simulink model "nonLin_Model_std_V2"  (R2023b)
settings: Solver=ode23t  StartTime=0.0  StopTime=Tend  FixedStep=Ts  MaxStep=0.002  RelTol=1e-3
InitFcn:
  | sysParam = load("sysParam.mat");
  | load('./zz_temp/controlletTypeToUse.mat')
undefined symbols (not defined in the file): C, sysID
libraries: slpidlib x12, cstblocks x2
(part 2 of 2)

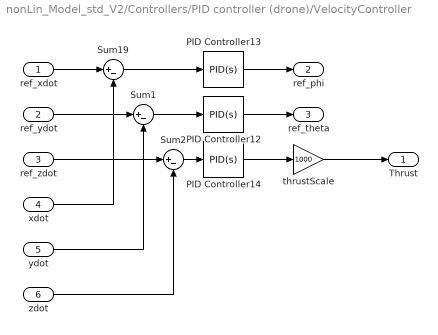
== system nonLin_Model_std_V2/Controllers/PID controller (drone)/VelocityController ==
  ref_xdot : Inport
  ref_ydot : Inport  Port=2
  ref_zdot : Inport  Port=3
  xdot : Inport  Port=4
  ydot : Inport  Port=5
  zdot : Inport  Port=6
  PID Controller12 : slpidlib/PID Controller  Controller=PID  Form=Parallel  TimeDomain=Continuous-time  UseExternalTs=off  SampleTime=-1  IntegratorMethod=Forward Euler  FilterMethod=Forward Euler  ControllerParametersSource=internal  P=C.vel.ydot.Kp  I=C.vel.ydot.Ki  UseKiTs=off  D=C.vel.ydot.Kd  N=100  UseFilter=on  TunerSelectOption=Transfer Function Based (PID Tuner App)  InitialConditionSource=internal  InitialConditionForIntegrator=0  InitialConditionForFilter=0  DifferentiatorICPrevScaledInput=0  ExternalReset=none  TrackingMode=off  Kt=1  LimitOutput=off  SatLimitsSource=internal  UpperSaturationLimit=inf  LowerSaturationLimit=-inf  LinearizeAsGain=on  AntiWindupMode=none  Kb=1  LimitIntegrator=off  UpperIntegratorSaturationLimit=inf  LowerIntegratorSaturationLimit=-inf  POutMin=[]  POutMax=[]  IOutMin=[]  IOutMax=[]  DOutMin=[]  DOutMax=[]  NOutMin=[]  NOutMax=[]  SumOutMin=[]  SumOutMax=[]  SaturationOutMin=[]  SaturationOutMax=[]  PParamMin=[]  PParamMax=[]  IParamMin=[]  IParamMax=[]  DParamMin=[]  DParamMax=[]  NParamMin=[]  NParamMax=[]  KbParamMin=[]  KbParamMax=[]  KtParamMin=[]  KtParamMax=[]  KbOutMin=[]  KbOutMax=[]  KtOutMin=[]  KtOutMax=[]  IntegratorOutMin=[]  IntegratorOutMax=[]  FilterOutMin=[]  FilterOutMax=[]  SumI1OutMin=[]  SumI1OutMax=[]  SumI2OutMin=[]  SumI2OutMax=[]  SumI3OutMin=[]  SumI3OutMax=[]  SumI4OutMin=[]  SumI4OutMax=[]  SumDOutMin=[]  SumDOutMax=[]  DifferentiatorOutMin=[]  DifferentiatorOutMax=[]  FilterDiffOutCoefMin=[]  FilterDiffOutCoefMax=[]  ReciprocalOutMin=[]  ReciprocalOutMax=[]  SumDenOutMin=[]  SumDenOutMax=[]  SumNumOutMin=[]  SumNumOutMax=[]  DivideOutMin=[]  DivideOutMax=[]  UdiffTsProdOutMin=[]  UdiffTsProdOutMax=[]  NTsProdOutMin=[]  NTsProdOutMax=[]  UintegralTsProdOutMin=[]  UintegralTsProdOutMax=[]  UngainTsProdOutMin=[]  UngainTsProdOutMax=[]  ClampingZeroOutDataTypeStr=Inherit: Inherit via back propagation  ClampingZeroOutMin=[]  ClampingZeroOutMax=[]  FilterDenConstantOutDataTypeStr=Inherit: Inherit via back propagation  FilterDenConstantOutMin=[]  FilterDenConstantOutMax=[]  PCopyOutDataTypeStr=Inherit: Inherit via back propagation  PCopyOutMin=[]  PCopyOutMax=[]  NCopyOutDataTypeStr=Inherit: Inherit via back propagation  NCopyOutMin=[]  NCopyOutMax=[]  IntegratorContinuousStateAttributes=''  IntegratorStateMustResolveToSignalObject=off  IntegratorRTWStateStorageClass=Auto  FilterContinuousStateAttributes=''  FilterStateMustResolveToSignalObject=off  FilterRTWStateStorageClass=Auto  ParallelPVariant=InternalParameters  IdealPVariant=Disabled  IVariant=InternalParameters  DVariant=InternalParameters  IntegratorVariant=Continuous  SatVariant=Disabled  AWVariant=Passthrough  PCopyVariant=Disabled  TRVariant=Disabled  FdbkBlocksVariant=Forward  IdealPFdbkVariant=Disabled  SatFdbkVariant=Disabled  DerivativeFilterVariant=ContFilter  NVariant=InternalParameters  NCopyVariant=Disabled  FilterICVariant=InternalICsFilter  IntegratorICVariant=InternalICs  ExternalResetVariant=Disabled  TRSumVariant=Passthrough  SumFdbkVariant=Disabled  SumVariant=Sum_PID  TsampFilterVariant=InternalTs  TsampNgainVariant=Passthrough  TsampIntegralVariant=Disabled_SignalSpec  ExternalSaturationOutDataTypeStr=Inherit: Same as second input
  PID Controller13 : slpidlib/PID Controller  Controller=PID  Form=Parallel  TimeDomain=Continuous-time  UseExternalTs=off  SampleTime=-1  IntegratorMethod=Forward Euler  FilterMethod=Forward Euler  ControllerParametersSource=internal  P=C.vel.xdot.Kp  I=C.vel.xdot.Ki  UseKiTs=off  D=C.vel.xdot.Kd  N=100  UseFilter=on  TunerSelectOption=Transfer Function Based (PID Tuner App)  InitialConditionSource=internal  InitialConditionForIntegrator=0  InitialConditionForFilter=0  DifferentiatorICPrevScaledInput=0  ExternalReset=none  TrackingMode=off  Kt=1  LimitOutput=off  SatLimitsSource=internal  UpperSaturationLimit=inf  LowerSaturationLimit=-inf  LinearizeAsGain=on  AntiWindupMode=none  Kb=1  LimitIntegrator=off  UpperIntegratorSaturationLimit=inf  LowerIntegratorSaturationLimit=-inf  POutMin=[]  POutMax=[]  IOutMin=[]  IOutMax=[]  DOutMin=[]  DOutMax=[]  NOutMin=[]  NOutMax=[]  SumOutMin=[]  SumOutMax=[]  SaturationOutMin=[]  SaturationOutMax=[]  PParamMin=[]  PParamMax=[]  IParamMin=[]  IParamMax=[]  DParamMin=[]  DParamMax=[]  NParamMin=[]  NParamMax=[]  KbParamMin=[]  KbParamMax=[]  KtParamMin=[]  KtParamMax=[]  KbOutMin=[]  KbOutMax=[]  KtOutMin=[]  KtOutMax=[]  IntegratorOutMin=[]  IntegratorOutMax=[]  FilterOutMin=[]  FilterOutMax=[]  SumI1OutMin=[]  SumI1OutMax=[]  SumI2OutMin=[]  SumI2OutMax=[]  SumI3OutMin=[]  SumI3OutMax=[]  SumI4OutMin=[]  SumI4OutMax=[]  SumDOutMin=[]  SumDOutMax=[]  DifferentiatorOutMin=[]  DifferentiatorOutMax=[]  FilterDiffOutCoefMin=[]  FilterDiffOutCoefMax=[]  ReciprocalOutMin=[]  ReciprocalOutMax=[]  SumDenOutMin=[]  SumDenOutMax=[]  SumNumOutMin=[]  SumNumOutMax=[]  DivideOutMin=[]  DivideOutMax=[]  UdiffTsProdOutMin=[]  UdiffTsProdOutMax=[]  NTsProdOutMin=[]  NTsProdOutMax=[]  UintegralTsProdOutMin=[]  UintegralTsProdOutMax=[]  UngainTsProdOutMin=[]  UngainTsProdOutMax=[]  ClampingZeroOutDataTypeStr=Inherit: Inherit via back propagation  ClampingZeroOutMin=[]  ClampingZeroOutMax=[]  FilterDenConstantOutDataTypeStr=Inherit: Inherit via back propagation  FilterDenConstantOutMin=[]  FilterDenConstantOutMax=[]  PCopyOutDataTypeStr=Inherit: Inherit via back propagation  PCopyOutMin=[]  PCopyOutMax=[]  NCopyOutDataTypeStr=Inherit: Inherit via back propagation  NCopyOutMin=[]  NCopyOutMax=[]  IntegratorContinuousStateAttributes=''  IntegratorStateMustResolveToSignalObject=off  IntegratorRTWStateStorageClass=Auto  FilterContinuousStateAttributes=''  FilterStateMustResolveToSignalObject=off  FilterRTWStateStorageClass=Auto  ParallelPVariant=InternalParameters  IdealPVariant=Disabled  IVariant=InternalParameters  DVariant=InternalParameters  IntegratorVariant=Continuous  SatVariant=Disabled  AWVariant=Passthrough  PCopyVariant=Disabled  TRVariant=Disabled  FdbkBlocksVariant=Forward  IdealPFdbkVariant=Disabled  SatFdbkVariant=Disabled  DerivativeFilterVariant=ContFilter  NVariant=InternalParameters  NCopyVariant=Disabled  FilterICVariant=InternalICsFilter  IntegratorICVariant=InternalICs  ExternalResetVariant=Disabled  TRSumVariant=Passthrough  SumFdbkVariant=Disabled  SumVariant=Sum_PID  TsampFilterVariant=InternalTs  TsampNgainVariant=Passthrough  TsampIntegralVariant=Disabled_SignalSpec  ExternalSaturationOutDataTypeStr=Inherit: Same as second input
  PID Controller14 : slpidlib/PID Controller  Controller=PID  Form=Parallel  TimeDomain=Continuous-time  UseExternalTs=off  SampleTime=-1  IntegratorMethod=Forward Euler  FilterMethod=Forward Euler  ControllerParametersSource=internal  P=C.vel.zdot.Kp  I=C.vel.zdot.Ki  UseKiTs=off  D=C.vel.zdot.Kd  N=100  UseFilter=on  TunerSelectOption=Transfer Function Based (PID Tuner App)  InitialConditionSource=internal  InitialConditionForIntegrator=0  InitialConditionForFilter=0  DifferentiatorICPrevScaledInput=0  ExternalReset=none  TrackingMode=off  Kt=1  LimitOutput=off  SatLimitsSource=internal  UpperSaturationLimit=inf  LowerSaturationLimit=-inf  LinearizeAsGain=on  AntiWindupMode=none  Kb=1  LimitIntegrator=off  UpperIntegratorSaturationLimit=inf  LowerIntegratorSaturationLimit=-inf  POutMin=[]  POutMax=[]  IOutMin=[]  IOutMax=[]  DOutMin=[]  DOutMax=[]  NOutMin=[]  NOutMax=[]  SumOutMin=[]  SumOutMax=[]  SaturationOutMin=[]  SaturationOutMax=[]  PParamMin=[]  PParamMax=[]  IParamMin=[]  IParamMax=[]  DParamMin=[]  DParamMax=[]  NParamMin=[]  NParamMax=[]  KbParamMin=[]  KbParamMax=[]  KtParamMin=[]  KtParamMax=[]  KbOutMin=[]  KbOutMax=[]  KtOutMin=[]  KtOutMax=[]  IntegratorOutMin=[]  IntegratorOutMax=[]  FilterOutMin=[]  FilterOutMax=[]  SumI1OutMin=[]  SumI1OutMax=[]  SumI2OutMin=[]  SumI2OutMax=[]  SumI3OutMin=[]  SumI3OutMax=[]  SumI4OutMin=[]  SumI4OutMax=[]  SumDOutMin=[]  SumDOutMax=[]  DifferentiatorOutMin=[]  DifferentiatorOutMax=[]  FilterDiffOutCoefMin=[]  FilterDiffOutCoefMax=[]  ReciprocalOutMin=[]  ReciprocalOutMax=[]  SumDenOutMin=[]  SumDenOutMax=[]  SumNumOutMin=[]  SumNumOutMax=[]  DivideOutMin=[]  DivideOutMax=[]  UdiffTsProdOutMin=[]  UdiffTsProdOutMax=[]  NTsProdOutMin=[]  NTsProdOutMax=[]  UintegralTsProdOutMin=[]  UintegralTsProdOutMax=[]  UngainTsProdOutMin=[]  UngainTsProdOutMax=[]  ClampingZeroOutDataTypeStr=Inherit: Inherit via back propagation  ClampingZeroOutMin=[]  ClampingZeroOutMax=[]  FilterDenConstantOutDataTypeStr=Inherit: Inherit via back propagation  FilterDenConstantOutMin=[]  FilterDenConstantOutMax=[]  PCopyOutDataTypeStr=Inherit: Inherit via back propagation  PCopyOutMin=[]  PCopyOutMax=[]  NCopyOutDataTypeStr=Inherit: Inherit via back propagation  NCopyOutMin=[]  NCopyOutMax=[]  IntegratorContinuousStateAttributes=''  IntegratorStateMustResolveToSignalObject=off  IntegratorRTWStateStorageClass=Auto  FilterContinuousStateAttributes=''  FilterStateMustResolveToSignalObject=off  FilterRTWStateStorageClass=Auto  ParallelPVariant=InternalParameters  IdealPVariant=Disabled  IVariant=InternalParameters  DVariant=InternalParameters  IntegratorVariant=Continuous  SatVariant=Disabled  AWVariant=Passthrough  PCopyVariant=Disabled  TRVariant=Disabled  FdbkBlocksVariant=Forward  IdealPFdbkVariant=Disabled  SatFdbkVariant=Disabled  DerivativeFilterVariant=ContFilter  NVariant=InternalParameters  NCopyVariant=Disabled  FilterICVariant=InternalICsFilter  IntegratorICVariant=InternalICs  ExternalResetVariant=Disabled  TRSumVariant=Passthrough  SumFdbkVariant=Disabled  SumVariant=Sum_PID  TsampFilterVariant=InternalTs  TsampNgainVariant=Passthrough  TsampIntegralVariant=Disabled_SignalSpec  ExternalSaturationOutDataTypeStr=Inherit: Same as second input
  Sum1 : Sum  Inputs=|+-
  Sum19 : Sum  Inputs=|+-
  Sum2 : Sum  Inputs=|+-
  thrustScale : Gain  Gain=1000
  Thrust : Outport
  ref_phi : Outport  Port=2
  ref_theta : Outport  Port=3
  wires:
  xdot/1 -> Sum19/2
  Sum19/1 -> PID Controller13/1
  Sum1/1 -> PID Controller12/1
  zdot/1 -> Sum2/2
  Sum2/1 -> PID Controller14/1
  ydot/1 -> Sum1/2
  ref_xdot/1 -> Sum19/1
  ref_ydot/1 -> Sum1/1
  ref_zdot/1 -> Sum2/1
  PID Controller14/1 -> thrustScale/1
  PID Controller12/1 -> ref_theta/1
  PID Controller13/1 -> ref_phi/1
  thrustScale/1 -> Thrust/1

== matlab function nonLin_Model_std_V2/non-linear model/MATLAB Function ==
  data: u input; dx output; x input; type input; sys_param2 parameter
function dx= nonLinDrone(u,x,type, sys_param2)
    m = sys_param2.m;
    I = sys_param2.I;
    g = sys_param2.g;
    % invI = inv(I);
    invI = sys_param2.inv_I;
    L = sys_param2.L;

    dx = zeros(12,1);
    
    % Angle states for easier use
    phi   = x(7); 
    theta = x(8); 
    psi   = x(9);
    p     = x(10); 
    q     = x(11); 
    r     = x(12);

    % Rotation matrix
    R = rotation_matrix(phi, theta, psi);

    % x and xdot definition
    dx(1:3,1) = [x(4); x(5); x(6)];
    dx(4:6,1) = 1/m*([0;0;-m*g]+R*[0;0;u(1)]);

    multiplication_matrix_pqr = ([1 sin(phi)*tan(theta) cos(phi)*tan(theta);0 cos(phi) -sin(phi);0 sin(phi)/cos(theta) cos(phi)/cos(theta)]);

    dx(7:9,1) = multiplication_matrix_pqr*[p;q;r];
    dx(10:12,1) = invI * ([u(2); u(3); u(4)] - cross([x(10);x(11);x(12)],I*[x(10);x(11);x(12)]));

    switch type
        case 1
            %F only
            dx([1:2 4:5 7:12]) = zeros(1,10);
        case 2
            %Mx only
            dx([1:6 8:9 11:12]) = zeros(1,10);
        case 3
            %My only
            dx([1:7 9:10 12]) = zeros(1,10);
        case 4
            %Mz only
            dx([1:8 10:11]) = zeros(1,10);
    end

function R = rotation_matrix(phi, theta, psi)
    R_x = [1 0 0; 0 cos(phi) -sin(phi); 0 sin(phi) cos(phi)];
    R_y = [cos(theta) 0 sin(theta); 0 1 0; -sin(theta) 0 cos(theta)];
    R_z = [cos(psi) -sin(psi) 0; sin(psi) cos(psi) 0; 0 0 1];

    R = R_z * R_y * R_x;
end
end

== matlab function nonLin_Model_std_V2/Controllers/PID controller (drone)/MATLAB Function ==
  data: rollRaw input; pitch_ref output; pitchRaw input; yawRad input; roll_ref output
function [pitch_ref,roll_ref] = fcn(rollRaw,pitchRaw,yawRad)

rp_limit = 20;

pitch_ref = -(rollRaw*cos(yawRad))-(pitchRaw*sin(yawRad));
roll_ref  = -(pitchRaw*cos(yawRad))+(rollRaw*sin(yawRad));

if pitch_ref>rp_limit
    pitch_ref = rp_limit;
elseif pitch_ref<-rp_limit
    pitch_ref = -rp_limit;
end
if roll_ref>rp_limit
    roll_ref = rp_limit;
elseif roll_ref<-rp_limit
    roll_ref = -rp_limit;
end

== matlab function nonLin_Model_std_V2/non-linear model/MATLAB Function2 ==
  data: input1 input; u output; input2 input; input3 input; input4 input
function u = fcn(input1,input2,input3,input4)

L = 0.048;% Distance from center of mass to rotors
% syms Thrust controlRoll controlPitch controlYaw
% 
% inputs = [Thrust;
%           controlRoll;
%           controlPitch;
%           controlYaw];

cmdi = [1 -0.5  0.5  1;
        1 -0.5 -0.5 -1;
        1  0.5 -0.5  1;
        1  0.5  0.5 -1]*[input1;input2;input3;input4];
% cmdi = [1 -2  2  1;
%         1 -2 -2 -1;
%         1  2 -2  1;
%         1  2  2 -1]*[input1;input2;input3;input4]

Kf2 = 2.130295e-11;
Kf1 = 1.032633e-6;
Kf0 = 5.484560e-4;

Km1 = 0.005964552;
Km0 = 1.563383;

Fi = Kf2*cmdi.^2+Kf1*cmdi+Kf0;
Mi = Km1*Fi+Km0;

u1 = sum(Fi);
% u2 = sqrt(2)*L*((Fi(1)+Fi(2))-(Fi(3)+Fi(4)));
% u3 = sqrt(2)*L*((Fi(2)+Fi(3))-(Fi(1)+Fi(4)));
u2 = L*(Fi(2)-Fi(4));
u3 = L*(Fi(3)-Fi(1));
u4 = Mi(1)-Mi(2)+Mi(3)-Mi(4);

u = [u1;u2;u3;u4];

end

== matlab function nonLin_Model_std_V2/Controllers/MPC controller/MPC controller ==
  data: x input; r_seq input; y0 input; u output
function u = MPC_Sparse_Controller(x, r_seq, y0)

u = testFUnc_MPC(x,zeros(15,1),y0,r_seq)



end
